simulink model "tseppid"  (R2020a)
settings: Solver=VariableStepAuto  StartTime=0.0  StopTime=360  RelTol=1e-3
undefined symbols (not defined in the file or in its folder): ini, qci, qgi, qwi
libraries: simulink x3
settings Model: Creator=sho  LastModifiedBy=sho
settings SolverCC: MaxConsecutiveMinStep=3

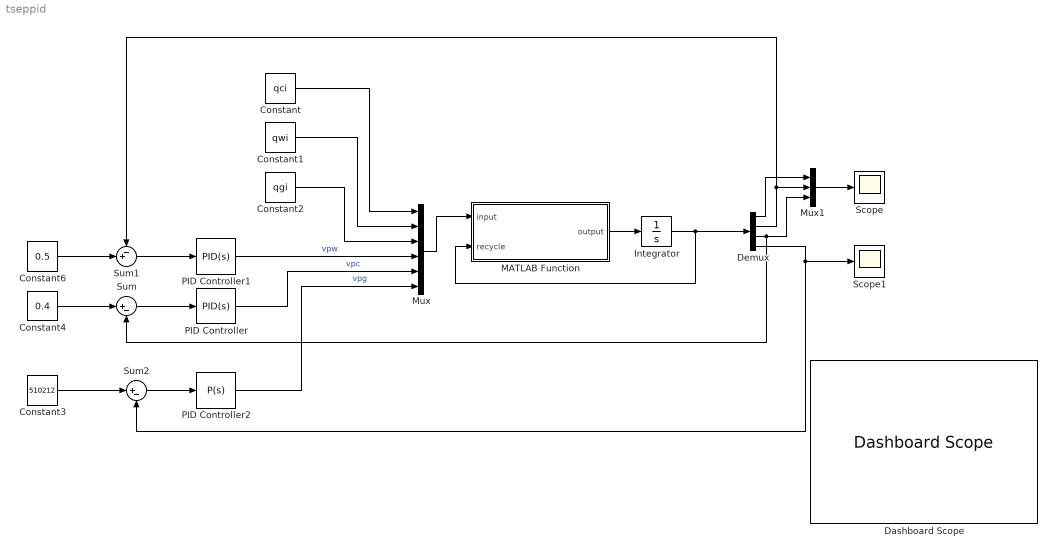
== system tseppid ==
  Constant : Constant  Value=qci
  Constant1 : Constant  Value=qwi
  Constant2 : Constant  Value=qgi
  Constant3 : Constant  Value=510212
  Constant4 : Constant  Value=0.4
  Constant6 : Constant  Value=0.5
  Dashboard Scope : DashboardScope
  Demux : Demux
  Integrator : Integrator  InitialCondition=ini
  MATLAB Function : MATLAB Function  TreatAsAtomicUnit=on
  Mux : Mux  Inputs=6
  Mux1 : Mux  Inputs=3
  PID Controller : simulink/Continuous/PID Controller  Controller=PID  Form=Parallel  TimeDomain=Continuous-time  UseExternalTs=off  SampleTime=-1  IntegratorMethod=Forward Euler  FilterMethod=Forward Euler  ControllerParametersSource=internal  P=-15  I=-1  D=0  UseFilter=on  N=100  TunerSelectOption=Transfer Function Based (PID Tuner App)  InitialConditionSource=internal  InitialConditionForIntegrator=0  InitialConditionForFilter=0  DifferentiatorICPrevScaledInput=0  ExternalReset=none  TrackingMode=off  Kt=1  LimitOutput=on  UpperSaturationLimit=1  LowerSaturationLimit=0  LinearizeAsGain=on  AntiWindupMode=none  Kb=1  POutMin=[]  POutMax=[]  IOutMin=[]  IOutMax=[]  DOutMin=[]  DOutMax=[]  NOutMin=[]  NOutMax=[]  SumOutMin=[]  SumOutMax=[]  SaturationOutMin=[]  SaturationOutMax=[]  PParamMin=[]  PParamMax=[]  IParamMin=[]  IParamMax=[]  DParamMin=[]  DParamMax=[]  NParamMin=[]  NParamMax=[]  KbParamMin=[]  KbParamMax=[]  KtParamMin=[]  KtParamMax=[]  KbOutMin=[]  KbOutMax=[]  KtOutMin=[]  KtOutMax=[]  IntegratorOutMin=[]  IntegratorOutMax=[]  FilterOutMin=[]  FilterOutMax=[]  SumI1OutMin=[]  SumI1OutMax=[]  SumI2OutMin=[]  SumI2OutMax=[]  SumI3OutMin=[]  SumI3OutMax=[]  SumI4OutMin=[]  SumI4OutMax=[]  SumDOutMin=[]  SumDOutMax=[]  DifferentiatorOutMin=[]  DifferentiatorOutMax=[]  FilterDiffOutCoefMin=[]  FilterDiffOutCoefMax=[]  ReciprocalOutMin=[]  ReciprocalOutMax=[]  SumDenOutMin=[]  SumDenOutMax=[]  SumNumOutMin=[]  SumNumOutMax=[]  DivideOutMin=[]  DivideOutMax=[]  UdiffTsProdOutMin=[]  UdiffTsProdOutMax=[]  NTsProdOutMin=[]  NTsProdOutMax=[]  UintegralTsProdOutMin=[]  UintegralTsProdOutMax=[]  UngainTsProdOutMin=[]  UngainTsProdOutMax=[]  IntegratorContinuousStateAttributes=''  IntegratorStateMustResolveToSignalObject=off  IntegratorRTWStateStorageClass=Auto  FilterContinuousStateAttributes=''  FilterStateMustResolveToSignalObject=off  FilterRTWStateStorageClass=Auto  ParallelPVariant=InternalParameters  IdealPVariant=Disabled  IVariant=InternalParameters  DVariant=InternalParameters  IntegratorVariant=Continuous  SatVariant=Enabled  AWVariant=Passthrough  PCopyVariant=Disabled  TRVariant=Disabled  FdbkBlocksVariant=Forward  IdealPFdbkVariant=Disabled  SatFdbkVariant=Disabled  DerivativeFilterVariant=ContFilter  NVariant=InternalParameters  NCopyVariant=Disabled  FilterICVariant=InternalICsFilter  IntegratorICVariant=InternalICs  ExternalResetVariant=Disabled  TRSumVariant=Passthrough  SumFdbkVariant=Disabled  SumVariant=Sum_PID  TsampFilterVariant=InternalTs  TsampNgainVariant=Passthrough  TsampIntegralVariant=Passthrough
  PID Controller1 : simulink/Continuous/PID Controller  Controller=PID  Form=Parallel  TimeDomain=Continuous-time  UseExternalTs=off  SampleTime=-1  IntegratorMethod=Forward Euler  FilterMethod=Forward Euler  ControllerParametersSource=internal  P=-15  I=-1  D=0  UseFilter=on  N=100  TunerSelectOption=Transfer Function Based (PID Tuner App)  InitialConditionSource=internal  InitialConditionForIntegrator=0  InitialConditionForFilter=0  DifferentiatorICPrevScaledInput=0  ExternalReset=none  TrackingMode=off  Kt=1  LimitOutput=on  UpperSaturationLimit=1  LowerSaturationLimit=0  LinearizeAsGain=on  AntiWindupMode=none  Kb=1  POutMin=[]  POutMax=[]  IOutMin=[]  IOutMax=[]  DOutMin=[]  DOutMax=[]  NOutMin=[]  NOutMax=[]  SumOutMin=[]  SumOutMax=[]  SaturationOutMin=[]  SaturationOutMax=[]  PParamMin=[]  PParamMax=[]  IParamMin=[]  IParamMax=[]  DParamMin=[]  DParamMax=[]  NParamMin=[]  NParamMax=[]  KbParamMin=[]  KbParamMax=[]  KtParamMin=[]  KtParamMax=[]  KbOutMin=[]  KbOutMax=[]  KtOutMin=[]  KtOutMax=[]  IntegratorOutMin=[]  IntegratorOutMax=[]  FilterOutMin=[]  FilterOutMax=[]  SumI1OutMin=[]  SumI1OutMax=[]  SumI2OutMin=[]  SumI2OutMax=[]  SumI3OutMin=[]  SumI3OutMax=[]  SumI4OutMin=[]  SumI4OutMax=[]  SumDOutMin=[]  SumDOutMax=[]  DifferentiatorOutMin=[]  DifferentiatorOutMax=[]  FilterDiffOutCoefMin=[]  FilterDiffOutCoefMax=[]  ReciprocalOutMin=[]  ReciprocalOutMax=[]  SumDenOutMin=[]  SumDenOutMax=[]  SumNumOutMin=[]  SumNumOutMax=[]  DivideOutMin=[]  DivideOutMax=[]  UdiffTsProdOutMin=[]  UdiffTsProdOutMax=[]  NTsProdOutMin=[]  NTsProdOutMax=[]  UintegralTsProdOutMin=[]  UintegralTsProdOutMax=[]  UngainTsProdOutMin=[]  UngainTsProdOutMax=[]  IntegratorContinuousStateAttributes=''  IntegratorStateMustResolveToSignalObject=off  IntegratorRTWStateStorageClass=Auto  FilterContinuousStateAttributes=''  FilterStateMustResolveToSignalObject=off  FilterRTWStateStorageClass=Auto  ParallelPVariant=InternalParameters  IdealPVariant=Disabled  IVariant=InternalParameters  DVariant=InternalParameters  IntegratorVariant=Continuous  SatVariant=Enabled  AWVariant=Passthrough  PCopyVariant=Disabled  TRVariant=Disabled  FdbkBlocksVariant=Forward  IdealPFdbkVariant=Disabled  SatFdbkVariant=Disabled  DerivativeFilterVariant=ContFilter  NVariant=InternalParameters  NCopyVariant=Disabled  FilterICVariant=InternalICsFilter  IntegratorICVariant=InternalICs  ExternalResetVariant=Disabled  TRSumVariant=Passthrough  SumFdbkVariant=Disabled  SumVariant=Sum_PID  TsampFilterVariant=InternalTs  TsampNgainVariant=Passthrough  TsampIntegralVariant=Passthrough
  PID Controller2 : simulink/Continuous/PID Controller  Controller=P  Form=Parallel  TimeDomain=Continuous-time  UseExternalTs=off  SampleTime=-1  IntegratorMethod=Forward Euler  FilterMethod=Forward Euler  ControllerParametersSource=internal  P=-15  I=1  D=0  UseFilter=on  N=100  TunerSelectOption=Transfer Function Based (PID Tuner App)  InitialConditionSource=internal  InitialConditionForIntegrator=0  InitialConditionForFilter=0  DifferentiatorICPrevScaledInput=0  ExternalReset=none  TrackingMode=off  Kt=1  LimitOutput=on  UpperSaturationLimit=1  LowerSaturationLimit=0  LinearizeAsGain=on  AntiWindupMode=none  Kb=1  POutMin=[]  POutMax=[]  IOutMin=[]  IOutMax=[]  DOutMin=[]  DOutMax=[]  NOutMin=[]  NOutMax=[]  SumOutMin=[]  SumOutMax=[]  SaturationOutMin=[]  SaturationOutMax=[]  PParamMin=[]  PParamMax=[]  IParamMin=[]  IParamMax=[]  DParamMin=[]  DParamMax=[]  NParamMin=[]  NParamMax=[]  KbParamMin=[]  KbParamMax=[]  KtParamMin=[]  KtParamMax=[]  KbOutMin=[]  KbOutMax=[]  KtOutMin=[]  KtOutMax=[]  IntegratorOutMin=[]  IntegratorOutMax=[]  FilterOutMin=[]  FilterOutMax=[]  SumI1OutMin=[]  SumI1OutMax=[]  SumI2OutMin=[]  SumI2OutMax=[]  SumI3OutMin=[]  SumI3OutMax=[]  SumI4OutMin=[]  SumI4OutMax=[]  SumDOutMin=[]  SumDOutMax=[]  DifferentiatorOutMin=[]  DifferentiatorOutMax=[]  FilterDiffOutCoefMin=[]  FilterDiffOutCoefMax=[]  ReciprocalOutMin=[]  ReciprocalOutMax=[]  SumDenOutMin=[]  SumDenOutMax=[]  SumNumOutMin=[]  SumNumOutMax=[]  DivideOutMin=[]  DivideOutMax=[]  UdiffTsProdOutMin=[]  UdiffTsProdOutMax=[]  NTsProdOutMin=[]  NTsProdOutMax=[]  UintegralTsProdOutMin=[]  UintegralTsProdOutMax=[]  UngainTsProdOutMin=[]  UngainTsProdOutMax=[]  IntegratorContinuousStateAttributes=''  IntegratorStateMustResolveToSignalObject=off  IntegratorRTWStateStorageClass=Auto  FilterContinuousStateAttributes=''  FilterStateMustResolveToSignalObject=off  FilterRTWStateStorageClass=Auto  ParallelPVariant=InternalParameters  IdealPVariant=Disabled  IVariant=Disabled  DVariant=Disabled  IntegratorVariant=Disabled  SatVariant=Enabled  AWVariant=Disabled  PCopyVariant=Disabled  TRVariant=Disabled  FdbkBlocksVariant=Forward  IdealPFdbkVariant=Disabled  SatFdbkVariant=Disabled  DerivativeFilterVariant=Disabled  NVariant=Disabled  NCopyVariant=Disabled_SignalSpec  FilterICVariant=Disabled  IntegratorICVariant=Disabled  ExternalResetVariant=Disabled  TRSumVariant=Passthrough  SumFdbkVariant=Disabled  SumVariant=Passthrough_P  TsampFilterVariant=InternalTs  TsampNgainVariant=Passthrough  TsampIntegralVariant=Disabled_SignalSpec
  Scope : Scope
  Scope1 : Scope
  Sum : Sum  Inputs=|+-
  Sum1 : Sum  Inputs=-+|
  Sum2 : Sum  Inputs=|+-
  wires:
  Mux/1 -> MATLAB Function/1(input)
  Constant/1 -> Mux/1
  Constant1/1 -> Mux/2
  MATLAB Function/1(output) -> Integrator/1
  Integrator/1 -> Demux/1, MATLAB Function/2(recycle)
  Constant2/1 -> Mux/3
  PID Controller1/1 -> Mux/4  "vpw"
  PID Controller/1 -> Mux/5  "vpc"
  Demux/1 -> Mux1/1
  Demux/2 -> Sum1/1, Mux1/2
  Demux/3 -> Mux1/3, Sum/2
  Mux1/1 -> Scope/1
  Demux/4 -> Sum2/2, Scope1/1
  Sum/1 -> PID Controller/1
  Constant4/1 -> Sum/1
  Constant6/1 -> Sum1/2
  Sum1/1 -> PID Controller1/1
  PID Controller2/1 -> Mux/6  "vpg"
  Sum2/1 -> PID Controller2/1
  Constant3/1 -> Sum2/1

== matlab function tseppid/MATLAB Function ==
  data: input input size=6; output output; recycle input size=4; const parameter
function output = tseptmodel(input,recycle,const)
%% Predefined parameters and constants

% Inputs
qci = input(1);         % Inflow of oil             [m3/s]
qwi = input(2);         % Inflow of water           [m3/s]
qgi = input(3);         % Inflow of gasr            [m3/s]
vpw = input(4);         % Fraq. opening VA          [adm]
vpc = input(5);         % Fraq. opening VB          [adm]
vpg = input(6);         % Fraq. opening VC          [adm]

% Geometric parameters
D = const(1);           % Separator's diameter      [m]
La = const(2);          % Length A section          [m]
Lb = const(3);          % Length B section          [m]
hs = const(4);          % Weir height               [m]
% Control parameters
kw = const(5);          % Water valve const.        [m3/s Pa^0.5]
poa = const(6);         % Outside pressure valve A  [Pa]
kc = const(7);          % Oil valve const.          [m3/s Pa^0.5]
pob = const(8);         % Outside pressure valve B  [Pa]
kg = const(9);          % Gas valve coef.           [m3/s Pa^0.5]
pog = const(10);        % Outside pressure valve C  [Pa]
% Fluid properties
rhoc = const(11);       % Oil density               [kg/m3]
gc = const(12);         % Oil Specific gravity      [adm]
rhow = const(13);       % Water density             [kg/m3]
gw = const(14);         % Water Specific gravity    [adm]
mg = const(15);         % Gas molar mass            [g/mol]
mair = const(16);       % Air molar mass            [g/mol]
% Physical constants
g = const(17);          % Gravity constant          [m/s2]
T = const(18);          % Temperature               [K]

% Recycle signals
hc = recycle(1);        % Prior iter. level hc      [m]
hw = recycle(2);        % Prior iter. level hw      [m]
hb = recycle(3);        % Prior iter. level hb      [m]
pg = recycle(4);        % Prior iter. pressure pg   [Pa]

%% Precalculated parameters

% Total volume separator
 vt = hemivolt(La,Lb,D);

% Oil level
 ha = hc+hw;

% Oil outlflow from Oil/water separator system
 if ha <= hs
    qca = 0;
 else
    % Weir equation (number) from Perry's Chemical Engineering Handbok
    qca = 0.415*(D-0.2*(ha-hs))*((ha-hs)^(1.5))*sqrt(2*g);
 end
 
 % Water outflow from Oil/water separator system
 qwo = kw*vpw*sqrt((pg+rhoc*g*hc+rhow*g*hw-poa)/gw);
 
 % Oil outflow from Oil collector system
 qcb = kc*vpc*sqrt((pg+rhoc*g*hb-pob)/gc);

 % Gas outflow from Gas system
 qgo = kg*vpg*sqrt(((pg-pog)*(pg+pog)*(T)*(mg/mair))/(pg^2));
 
 % Volume calculations
 va = hemivol(ha,La,D);
 vb = hemivol(hb,Lb,D);
 
%% Mass balances

% Fluid level ha - Oil/water separator system 
% dha = (qci+qwi-qca-qwo)/hemihead(ha,La,D);
dhc = (qci-qca)/hemihead(hc,La,D);

% Water level hw - Oil/water separator system 
dhw = (qwi-qwo)/hemihead(hw,La,D);

% Oil level hb - Oil collector system
dhb = (qca-qcb)/hemihead(hb,Lb,D);

disp(hw+hc);

% Pressure of gass Pg
dpg = pg*(qci+qwi-qwo-qcb+qgi-qgo)/(vt-va-vb);


output = [dhc; dhw; dhb; dpg];
